simulink model "EKF_Sim"  (R2023b)
settings: Solver=ode4  StartTime=t(1)  StopTime=t(end)  FixedStep=dt  RelTol=1e-3
values from neighbouring files (symbols this model uses):
  xInitial = [initial_conditions ... (first row only)    [gois09_simulink.m]    (also in hilaire07martinez_simulink.m = initial_conditions(1:2); jewett99_simulink.m = initial_conditions(1:2); ryzhii14_simulink.m; sinoatrial_simulink.m = initial_conditions)
undefined symbols (not defined in the file or in its folder): F, Q, R
settings Model: Creator=chukw  LastModifiedBy=chukw

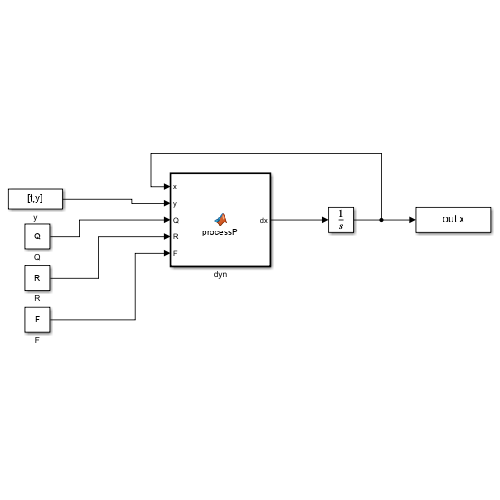
[thumbnail: Simulink's stored preview of the top-level diagram]
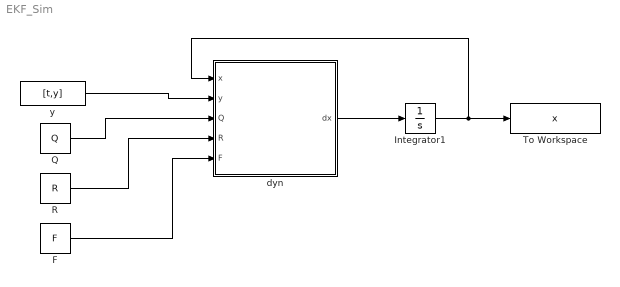
== system EKF_Sim ==
  F : Constant  Value=F
  Integrator1 : Integrator  InitialCondition=xInitial
  Q : Constant  Value=Q
  R : Constant  Value=R
  To Workspace : ToWorkspace  VariableName=x  SampleTime=-1
  dyn : MATLAB Function  TreatAsAtomicUnit=on
  y : FromWorkspace  VariableName=[t,y]
  wires:
  y/1 -> dyn/2(y)
  Integrator1/1 -> dyn/1(x), To Workspace/1
  dyn/1(dx) -> Integrator1/1
  F/1 -> dyn/5(F)
  R/1 -> dyn/4(R)
  Q/1 -> dyn/3(Q)

== matlab function EKF_Sim/dyn ==
  data: x input; y input; dx output; Q input; R input; F input
function dx = processP(x, y, Q, R, F)
    w = 2*pi/24;
    numStates = 7;

    P_vec = x(numStates+1:end);
    P = reshape(P_vec, numStates, numStates);

    yHat = [(x(1)) + x(3); (x(6)*x(1)) + (x(7)*x(2)/w) + x(4)];
    yTilde = y - yHat;

    H = [1, 0, 1, 0, 0, 0, 0;
         x(6), x(7)/w, 0, 1, 0, x(1), x(2)/w];
    K = P*H'/R;

    dx = zeros(numStates + (numStates^2), 1);
    dx(1) = x(2) + K(1, :)*yTilde;
    dx(2) = (-(w^2)*x(1)) + K(2, :)*yTilde;
    dx(3:7) = K(3:end, :)*yTilde;

    dP = F*P + P*F' - K*H*P + Q;
    dx(numStates+1:end) = dP(:);
end
